simulink subsystem "Controlobject"  (R2023a)
settings: Solver=VariableStepAuto  StartTime=0.0  StopTime=10.0  RelTol=1e-3
settings Model: Creator=stude  LastModifiedBy=hidra

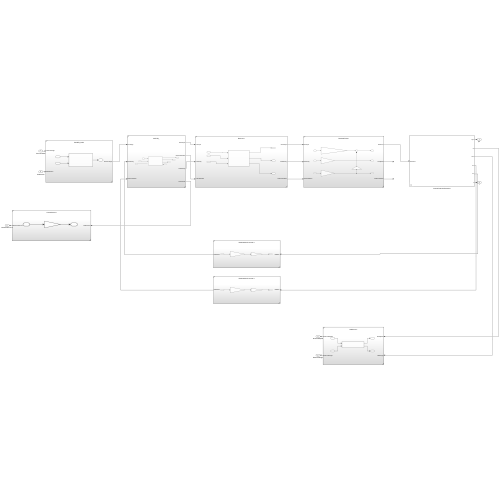
[thumbnail: Simulink's stored preview of the top-level diagram]
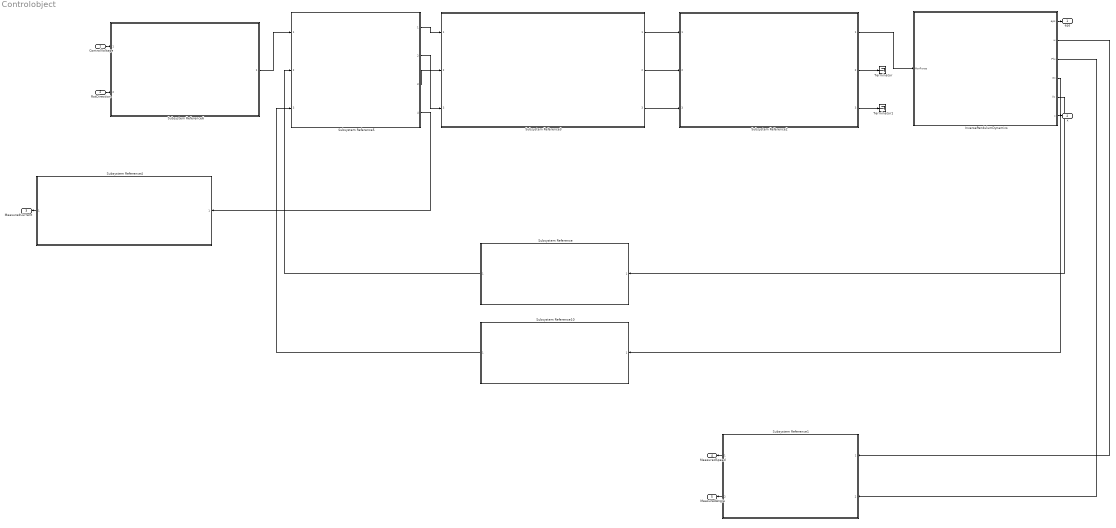
== system Controlobject ==
  ControlVoltage : Inport
  RotDirection : Inport  Port=2
  InversePendulumDynamics : Subsystem  mask{M=0.2, mr=0.1, l=1, g=9.81}
      mask prompts: M "Base mass"; mr "Rod mass"; l "Rod length"; g "Acceleration of gravity"
  Subsystem Reference : Subsystem  ReferencedSubsystem=BackwardAccConverter1
  Subsystem Reference1 : Subsystem  ReferencedSubsystem=HallSensor1
  Subsystem Reference10 : Subsystem  ReferencedSubsystem=BackwardAccConverter1
  Subsystem Reference2 : Subsystem  ReferencedSubsystem=RackandPinion1
  Subsystem Reference3 : Subsystem  ReferencedSubsystem=Reductor1
  Subsystem Reference4 : Subsystem  ReferencedSubsystem=CurrentSensor1
  Subsystem Reference5 : Subsystem  ReferencedSubsystem=MOTOR_
  Subsystem Reference6 : Subsystem  ReferencedSubsystem=POWER_GAIN
  Terminator : Terminator
  Terminator1 : Terminator
  eps : Outport
  x : Outport  Port=2
  MeasuredCurrent : Outport  Port=3
  MeasuredSpeed : Outport  Port=4
  MeasuredAngle : Outport  Port=5
  wires:
  Subsystem Reference5/3 -> Subsystem Reference3/2
  Subsystem Reference1/2 -> MeasuredAngle/1
  ControlVoltage/1 -> Subsystem Reference6/1
  Subsystem Reference4/1 -> MeasuredCurrent/1
  InversePendulumDynamics/1(eps) -> eps/1
  Subsystem Reference2/3 -> Terminator1/1
  InversePendulumDynamics/2(w) -> Subsystem Reference1/1
  Subsystem Reference5/4 -> Subsystem Reference4/1
  Subsystem Reference5/1 -> Subsystem Reference3/1
  InversePendulumDynamics/6(x) -> x/1
  Subsystem Reference3/2 -> Subsystem Reference2/2
  Subsystem Reference1/1 -> MeasuredSpeed/1
  Subsystem Reference/1 -> Subsystem Reference5/2
  Subsystem Reference3/1 -> Subsystem Reference2/1
  Subsystem Reference6/1 -> Subsystem Reference5/1
  InversePendulumDynamics/3(Phi) -> Subsystem Reference1/2
  Subsystem Reference5/2 -> Subsystem Reference3/3
  InversePendulumDynamics/4(ax) -> Subsystem Reference10/1
  Subsystem Reference3/3 -> Subsystem Reference2/3
  Subsystem Reference2/1 -> InversePendulumDynamics/1(HorForce)
  Subsystem Reference2/2 -> Terminator/1
  InversePendulumDynamics/5(Vx) -> Subsystem Reference/1
  Subsystem Reference10/1 -> Subsystem Reference5/3
  RotDirection/1 -> Subsystem Reference6/2

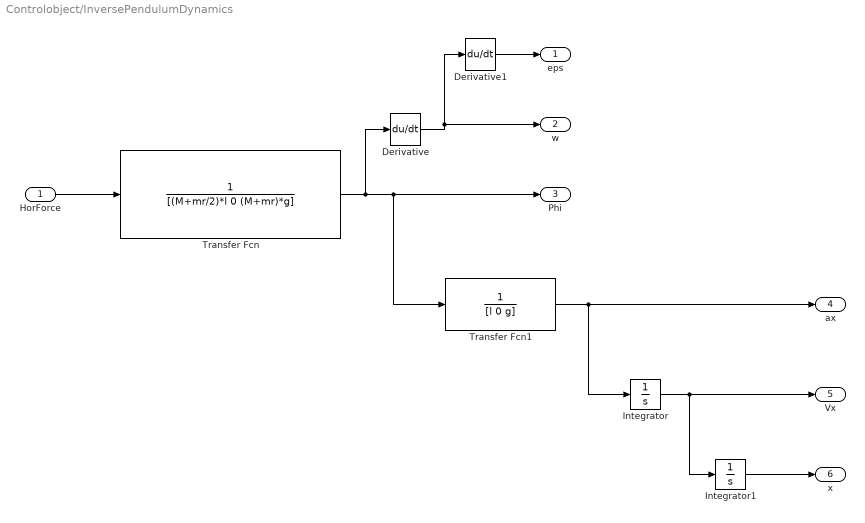
== system Controlobject/InversePendulumDynamics ==
  HorForce : Inport
  Derivative : Derivative
  Derivative1 : Derivative
  Integrator : Integrator
  Integrator1 : Integrator
  Transfer Fcn : TransferFcn  Denominator=[(M+mr/2)*l 0 (M+mr)*g]
  Transfer Fcn1 : TransferFcn  Denominator=[l 0 g]
  eps : Outport
  w : Outport  Port=2
  Phi : Outport  Port=3
  ax : Outport  Port=4
  Vx : Outport  Port=5
  x : Outport  Port=6
  wires:
  Integrator1/1 -> x/1
  HorForce/1 -> Transfer Fcn/1
  Derivative1/1 -> eps/1
  Integrator/1 -> Vx/1, Integrator1/1
  Transfer Fcn/1 -> Phi/1, Transfer Fcn1/1, Derivative/1
  Derivative/1 -> w/1, Derivative1/1
  Transfer Fcn1/1 -> ax/1, Integrator/1
